simulink model "DC_microgrid_sliding_mode_control_NIKHIL_TYAGI"  (R2023b)
settings: Solver=VariableStepAuto  StartTime=0.0  StopTime=5  RelTol=1e-3
undefined symbols (not defined in the file): Ion, Lithium
libraries: spsFirstOrderFilterLib x19, spsCurrentMeasurementLib x11, spsSeriesRLCBranchLib x10, spsIGBTDiodeLib x4, spsVoltageMeasurementLib x4, spsPWMGeneratorDCDCLib x3, slpidlib x2, spsStairGeneratorLib x2, spsBatteryLib x1, spsDiodeLib x1, spsGroundLib x1, spsIGBTLib x1
settings Model: Creator=tyagi  LastModifiedBy=tyagi_av27qbo
settings OptimizationCC: ReuseModelBlockBuffer=off

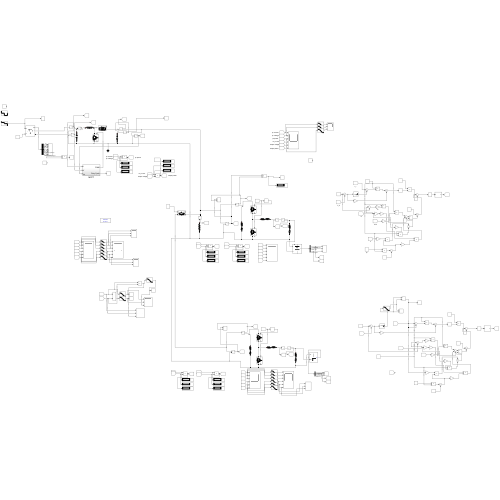
[thumbnail: Simulink's stored preview of the top-level diagram]
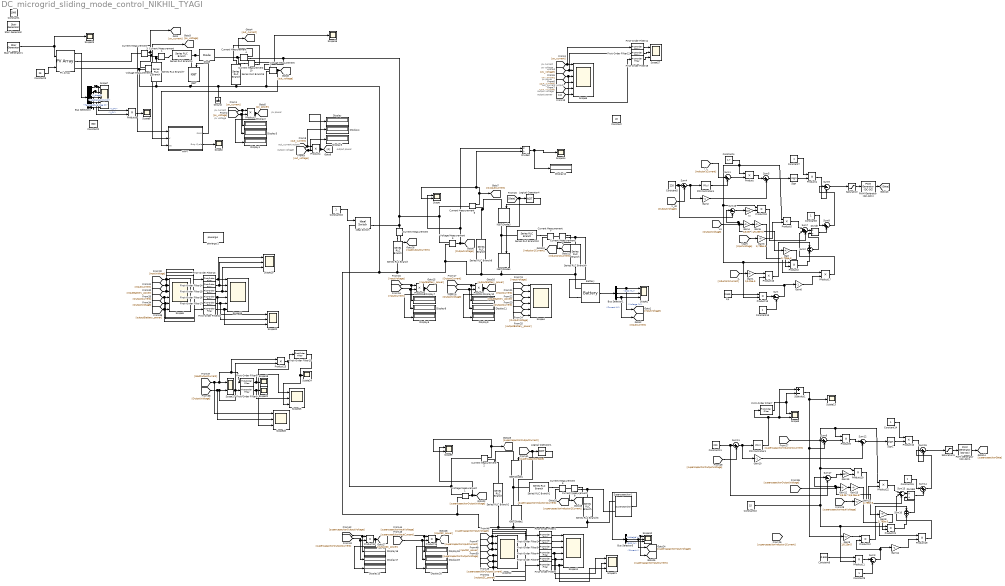
== system DC_microgrid_sliding_mode_control_NIKHIL_TYAGI ==
  note: pv power
  note: pv current
  note: out_current output
  note: pv voltage
  note: output voltage
  note: out_current output
  note: pv voltage
  note: pv power
  note: output voltage
  note: pv current
  note: output power
  note: output power
  Battery : spsBatteryLib/Battery  BatType=Lithium-Ion  ShowTempParam=off  ThermalPreset=no  ShowAgeParam=off  NomV=150  NomQ=15  SOC=100  Batt_Tr=30  PresetModel=on  MaxQ=15  MinV=112.5  FullV=174.5981  Dis_rate=6.5217  R=0.1  Normal_OP=13.5652  expZone="[162.0579     0.7369565]"  current=[6.5 13 32.5]  Units=Time  Tci=20  NomT=20  T2=-30  MaxQ2=4.8  FullV2=7.1  Normal_OP2=5.655  expZone2="[6.58           1]"  Rca=0.6  ti=2000  Dp=0  Neq0=0  Tsim=1e6  Ta1=25  Qeol=5.4*0.9  Reol=0.013333*1.2  Char_age=[2.3478, 3]  Dis_age=[2.3478, 10]  N1=1500  N2=10500  N3=1000  N4=1400  Ta2=45  N5=950
  Bus Selector1 : BusSelector  OutputSignals=Voltage (V),SOC (%),Current (A)
  Bus Selector2 : BusSelector  OutputSignals=V_PV,I_PV,I_diode,Irradiance (W/m2),Temperature (deg C)
  Bus Selector5 : BusSelector  OutputSignals=Current I,Voltage V,SOC %
  Constant : Constant  Value=40
  Constant1 : Constant  Value=1000
  Constant10 : Constant  Value=15
  Constant11 : Constant  Value=220
  Constant{7..9,13..16} (7 alike) : Constant
  Constant2 : Constant  Value=800
  Constant3 : Constant  Value=25
  Constant4 : Constant  Value=1.7
  Constant5 : Constant  Value=220
  Constant6 : Constant  Value=0.646
  Current Measurement{,1..10} (11 alike) : spsCurrentMeasurementLib/Current Measurement  PhasorSimulation=off  OutputType=Complex  PSBequivalent=0
  Diode : spsDiodeLib/Diode  Ron=0.001  Lon=0  Vf=0.8  IC=0  UseSnubber=0  Rs=500  Cs=250e-9  Measurements=on
  Display{,1..12,15..20} (19 alike) : Display
  Divide : Product  Inputs=*/
  Divide1 : Product  Inputs=*/
  Divide2 : Product  Inputs=*/
  First-Order Filter{1..6,8..19} (18 alike) : spsFirstOrderFilterLib/First-Order Filter  FilterType=Lowpass  Tc=10e-3  Ts=0  Initialize=on  Vac_Init=[0, 0, 60]  Vdc_Init=0  PlotResponse=off  FreqRange="[0,  200,  1]"
  First-Order Filter7 : spsFirstOrderFilterLib/First-Order Filter  FilterType=Lowpass  Tc=10e-3  Ts=0  Initialize=on  Vac_Init=[0, 0, 0]  Vdc_Init=0  PlotResponse=off  FreqRange="[0,  200,  1]"
  From13 : From
  Gain{,3,8,11} (4 alike) : Gain  Gain=1/.795e-3
  Gain1 : Gain  Gain=1/5.25e-5
  Gain{2,6,10,14} (4 alike) : Gain  Gain=-1
  Gain12 : Gain  Gain=1/8.06
  Gain13 : Gain  Gain=(1/5.25e-5)
  Gain15 : Gain  Gain=227
  Gain4 : Gain  Gain=1/8.06
  Gain5 : Gain  Gain=(1/5.25e-5)
  Gain9 : Gain  Gain=1/5.25e-5
  Goto9 : Goto
  Ground : spsGroundLib/Ground  LConnTagsString=a
  IGBT : spsIGBTLib/IGBT  Ron=0.001  Lon=0  Vf=1  Tf=1e-6  Tt=2e-6  IC=0  Rs=1e5  Cs=inf  Measurements=on
  IGBT/Diode{1..4} (4 alike) : spsIGBTDiodeLib/IGBT//Diode  Ron=1e-3  Rs=1e5  Cs=inf  Measurements=on
  Ideal Switch : spsIdealSwitchLib/Ideal Switch  Ron=0.001  Lon=0  IC=0  Rs=1e5  Cs=inf  Measurements=on
  Ki : Gain  Gain=227
  Kp : Constant  Value=0.646
  Logical Operator1 : Logic  Operator=NOT  AllPortsSameDT=off  OutDataTypeStr=boolean
  Logical Operator4 : Logic  Operator=NOT  AllPortsSameDT=off  OutDataTypeStr=boolean
  MPPT : Subsystem
  PID Controller1 : slpidlib/PID Controller  Controller=PI  Form=Parallel  TimeDomain=Continuous-time  UseExternalTs=off  SampleTime=-1  IntegratorMethod=Forward Euler  FilterMethod=Forward Euler  ControllerParametersSource=internal  P=0.646  I=227  UseKiTs=off  D=0  N=100  UseFilter=on  TunerSelectOption=Transfer Function Based (PID Tuner App)  InitialConditionSource=internal  InitialConditionForIntegrator=0  InitialConditionForFilter=0  DifferentiatorICPrevScaledInput=0  ExternalReset=none  TrackingMode=off  Kt=1  LimitOutput=on  SatLimitsSource=internal  UpperSaturationLimit=45  LowerSaturationLimit=0  LinearizeAsGain=on  AntiWindupMode=none  Kb=1  LimitIntegrator=off  UpperIntegratorSaturationLimit=inf  LowerIntegratorSaturationLimit=-inf  POutMin=[]  POutMax=[]  IOutMin=[]  IOutMax=[]  DOutMin=[]  DOutMax=[]  NOutMin=[]  NOutMax=[]  SumOutMin=[]  SumOutMax=[]  SaturationOutMin=[]  SaturationOutMax=[]  PParamMin=[]  PParamMax=[]  IParamMin=[]  IParamMax=[]  DParamMin=[]  DParamMax=[]  NParamMin=[]  NParamMax=[]  KbParamMin=[]  KbParamMax=[]  KtParamMin=[]  KtParamMax=[]  KbOutMin=[]  KbOutMax=[]  KtOutMin=[]  KtOutMax=[]  IntegratorOutMin=[]  IntegratorOutMax=[]  FilterOutMin=[]  FilterOutMax=[]  SumI1OutMin=[]  SumI1OutMax=[]  SumI2OutMin=[]  SumI2OutMax=[]  SumI3OutMin=[]  SumI3OutMax=[]  SumI4OutMin=[]  SumI4OutMax=[]  SumDOutMin=[]  SumDOutMax=[]  DifferentiatorOutMin=[]  DifferentiatorOutMax=[]  FilterDiffOutCoefMin=[]  FilterDiffOutCoefMax=[]  ReciprocalOutMin=[]  ReciprocalOutMax=[]  SumDenOutMin=[]  SumDenOutMax=[]  SumNumOutMin=[]  SumNumOutMax=[]  DivideOutMin=[]  DivideOutMax=[]  UdiffTsProdOutMin=[]  UdiffTsProdOutMax=[]  NTsProdOutMin=[]  NTsProdOutMax=[]  UintegralTsProdOutMin=[]  UintegralTsProdOutMax=[]  UngainTsProdOutMin=[]  UngainTsProdOutMax=[]  ClampingZeroOutDataTypeStr=Inherit: Inherit via back propagation  ClampingZeroOutMin=[]  ClampingZeroOutMax=[]  FilterDenConstantOutDataTypeStr=Inherit: Inherit via back propagation  FilterDenConstantOutMin=[]  FilterDenConstantOutMax=[]  PCopyOutDataTypeStr=Inherit: Inherit via back propagation  PCopyOutMin=[]  PCopyOutMax=[]  NCopyOutDataTypeStr=Inherit: Inherit via back propagation  NCopyOutMin=[]  NCopyOutMax=[]  IntegratorContinuousStateAttributes=''  IntegratorStateMustResolveToSignalObject=off  IntegratorRTWStateStorageClass=Auto  FilterContinuousStateAttributes=''  FilterStateMustResolveToSignalObject=off  FilterRTWStateStorageClass=Auto  ParallelPVariant=InternalParameters  IdealPVariant=Disabled  IVariant=InternalParameters  DVariant=Disabled  IntegratorVariant=Continuous  SatVariant=Enabled  AWVariant=Passthrough  PCopyVariant=Disabled  TRVariant=Disabled  FdbkBlocksVariant=Forward  IdealPFdbkVariant=Disabled  SatFdbkVariant=Disabled  DerivativeFilterVariant=Disabled  NVariant=Disabled  NCopyVariant=Disabled_SignalSpec  FilterICVariant=Disabled  IntegratorICVariant=InternalICs  ExternalResetVariant=Disabled  TRSumVariant=Passthrough  SumFdbkVariant=Disabled  SumVariant=Sum_PI  TsampFilterVariant=InternalTs  TsampNgainVariant=Passthrough  TsampIntegralVariant=Disabled_SignalSpec  ExternalSaturationOutDataTypeStr=Inherit: Same as second input
  PID Controller4 : slpidlib/PID Controller  Controller=PI  Form=Parallel  TimeDomain=Continuous-time  UseExternalTs=off  SampleTime=-1  IntegratorMethod=Forward Euler  FilterMethod=Forward Euler  ControllerParametersSource=internal  P=0.646  I=227  UseKiTs=off  D=0  N=100  UseFilter=on  TunerSelectOption=Transfer Function Based (PID Tuner App)  InitialConditionSource=internal  InitialConditionForIntegrator=0  InitialConditionForFilter=0  DifferentiatorICPrevScaledInput=0  ExternalReset=none  TrackingMode=off  Kt=1  LimitOutput=on  SatLimitsSource=internal  UpperSaturationLimit=45  LowerSaturationLimit=0  LinearizeAsGain=on  AntiWindupMode=none  Kb=1  LimitIntegrator=off  UpperIntegratorSaturationLimit=inf  LowerIntegratorSaturationLimit=-inf  POutMin=[]  POutMax=[]  IOutMin=[]  IOutMax=[]  DOutMin=[]  DOutMax=[]  NOutMin=[]  NOutMax=[]  SumOutMin=[]  SumOutMax=[]  SaturationOutMin=[]  SaturationOutMax=[]  PParamMin=[]  PParamMax=[]  IParamMin=[]  IParamMax=[]  DParamMin=[]  DParamMax=[]  NParamMin=[]  NParamMax=[]  KbParamMin=[]  KbParamMax=[]  KtParamMin=[]  KtParamMax=[]  KbOutMin=[]  KbOutMax=[]  KtOutMin=[]  KtOutMax=[]  IntegratorOutMin=[]  IntegratorOutMax=[]  FilterOutMin=[]  FilterOutMax=[]  SumI1OutMin=[]  SumI1OutMax=[]  SumI2OutMin=[]  SumI2OutMax=[]  SumI3OutMin=[]  SumI3OutMax=[]  SumI4OutMin=[]  SumI4OutMax=[]  SumDOutMin=[]  SumDOutMax=[]  DifferentiatorOutMin=[]  DifferentiatorOutMax=[]  FilterDiffOutCoefMin=[]  FilterDiffOutCoefMax=[]  ReciprocalOutMin=[]  ReciprocalOutMax=[]  SumDenOutMin=[]  SumDenOutMax=[]  SumNumOutMin=[]  SumNumOutMax=[]  DivideOutMin=[]  DivideOutMax=[]  UdiffTsProdOutMin=[]  UdiffTsProdOutMax=[]  NTsProdOutMin=[]  NTsProdOutMax=[]  UintegralTsProdOutMin=[]  UintegralTsProdOutMax=[]  UngainTsProdOutMin=[]  UngainTsProdOutMax=[]  ClampingZeroOutDataTypeStr=Inherit: Inherit via back propagation  ClampingZeroOutMin=[]  ClampingZeroOutMax=[]  FilterDenConstantOutDataTypeStr=Inherit: Inherit via back propagation  FilterDenConstantOutMin=[]  FilterDenConstantOutMax=[]  PCopyOutDataTypeStr=Inherit: Inherit via back propagation  PCopyOutMin=[]  PCopyOutMax=[]  NCopyOutDataTypeStr=Inherit: Inherit via back propagation  NCopyOutMin=[]  NCopyOutMax=[]  IntegratorContinuousStateAttributes=''  IntegratorStateMustResolveToSignalObject=off  IntegratorRTWStateStorageClass=Auto  FilterContinuousStateAttributes=''  FilterStateMustResolveToSignalObject=off  FilterRTWStateStorageClass=Auto  ParallelPVariant=InternalParameters  IdealPVariant=Disabled  IVariant=InternalParameters  DVariant=Disabled  IntegratorVariant=Continuous  SatVariant=Enabled  AWVariant=Passthrough  PCopyVariant=Disabled  TRVariant=Disabled  FdbkBlocksVariant=Forward  IdealPFdbkVariant=Disabled  SatFdbkVariant=Disabled  DerivativeFilterVariant=Disabled  NVariant=Disabled  NCopyVariant=Disabled_SignalSpec  FilterICVariant=Disabled  IntegratorICVariant=InternalICs  ExternalResetVariant=Disabled  TRSumVariant=Passthrough  SumFdbkVariant=Disabled  SumVariant=Sum_PI  TsampFilterVariant=InternalTs  TsampNgainVariant=Passthrough  TsampIntegralVariant=Disabled_SignalSpec  ExternalSaturationOutDataTypeStr=Inherit: Same as second input
  PV Array : spsPVArrayLib/PV Array  Npar=8  Nser=2  PlotType=array @ 25 deg.C & specified irradiances  S_vec="[ 1000  500  100 ]"  Temp_C_vec="[ 45 25  ]"  ModuleName=SunPower SPR-E19-310-COM  PlotWhenSelected=off  Pm=310.149  Ncell=96  Voc=64.4  Isc=6.05  Vm=54.7  Im=5.67  beta_Voc_pc=-0.2727  alpha_Isc_pc=0.061736  beta_Voc=-0.17562  alpha_Isc=0.003735  IL=6.0753  I0=6.4157e-12  nI=0.94792  Rsh=341.5455  Rs=0.40157  RobustModel=off  RobustCellTemperature=313.3991  BAL=off  Tc=1e-6  Tfilter=5e-5
  PWM Generator (DC-DC)1 : spsPWMGeneratorDCDCLib/PWM Generator (DC-DC)  Fsw=15000  Ts=0
  PWM Generator (DC-DC)2 : spsPWMGeneratorDCDCLib/PWM Generator (DC-DC)  Fsw=15000  Ts=0
  Product{,1..23} (24 alike) : Product
  Saturation : Saturate  UpperLimit=1  LowerLimit=0
  Saturation1 : Saturate  UpperLimit=1  LowerLimit=0
  Scope{,3,9,17} (4 alike) : Scope  NumInputPorts=2
  Scope{1,10,19..21,25,27..28} (8 alike) : Scope  NumInputPorts=3
  Scope{4..6,11..12,15} (6 alike) : Scope  NumInputPorts=6
  Scope{2,8,13..14,16,18,22..24} (9 alike) : Scope
  Scope7 : Scope  NumInputPorts=5
  Series RLC Branch : spsSeriesRLCBranchLib/Series RLC Branch  LConnTagsString=__new0  RConnTagsString=__new0  BranchType=R  Resistance=8.06  Inductance=1e-3  SetiL0=off  InitialCurrent=0  Capacitance=1e-6  Setx0=off  InitialVoltage=0  Measurements=None
  Series RLC Branch1 : spsSeriesRLCBranchLib/Series RLC Branch  LConnTagsString=__new0  RConnTagsString=__new0  BranchType=RL  Resistance=0.0001  Inductance=.795e-3  SetiL0=off  InitialCurrent=0  Capacitance=1e-6  Setx0=off  InitialVoltage=0  Measurements=None
  Series RLC Branch10 : spsSeriesRLCBranchLib/Series RLC Branch  LConnTagsString=__new0  RConnTagsString=__new0  BranchType=RL  Resistance=0.0001  Inductance=.795e-3  SetiL0=off  InitialCurrent=0  Capacitance=1e-6  Setx0=off  InitialVoltage=0  Measurements=None
  Series RLC Branch2 : spsSeriesRLCBranchLib/Series RLC Branch  LConnTagsString=__new0  RConnTagsString=__new0  BranchType=RC  Resistance=.0001  Inductance=1e-3  SetiL0=off  InitialCurrent=0  Capacitance=1000e-6  Setx0=off  InitialVoltage=0  Measurements=None
  Series RLC Branch3 : spsSeriesRLCBranchLib/Series RLC Branch  LConnTagsString=__new0  RConnTagsString=__new0  BranchType=RC  Resistance=0.0001  Inductance=1e-3  SetiL0=off  InitialCurrent=0  Capacitance=4.44e-6  Setx0=off  InitialVoltage=0  Measurements=None
  Series RLC Branch4 : spsSeriesRLCBranchLib/Series RLC Branch  LConnTagsString=__new0  RConnTagsString=__new0  BranchType=L  Resistance=1  Inductance=.336e-3  SetiL0=off  InitialCurrent=0  Capacitance=1e-6  Setx0=off  InitialVoltage=0  Measurements=None
  Series RLC Branch6 : spsSeriesRLCBranchLib/Series RLC Branch  LConnTagsString=__new0  RConnTagsString=__new0  BranchType=C  Resistance=0.001  Inductance=1e-3  SetiL0=off  InitialCurrent=0  Capacitance=4000.31e-6  Setx0=off  InitialVoltage=0  Measurements=None
  Series RLC Branch7 : spsSeriesRLCBranchLib/Series RLC Branch  LConnTagsString=__new0  RConnTagsString=__new0  BranchType=C  Resistance=1e-3  Inductance=1e-3  SetiL0=off  InitialCurrent=0  Capacitance=1000e-6  Setx0=off  InitialVoltage=0  Measurements=None
  Series RLC Branch8 : spsSeriesRLCBranchLib/Series RLC Branch  LConnTagsString=__new0  RConnTagsString=__new0  BranchType=RC  Resistance=.0001  Inductance=1e-3  SetiL0=off  InitialCurrent=0  Capacitance=1000e-6  Setx0=off  InitialVoltage=0  Measurements=None
  Series RLC Branch9 : spsSeriesRLCBranchLib/Series RLC Branch  LConnTagsString=__new0  RConnTagsString=__new0  BranchType=RC  Resistance=0.0001  Inductance=1e-3  SetiL0=off  InitialCurrent=0  Capacitance=4.44e-6  Setx0=off  InitialVoltage=0  Measurements=None
  Sign : Signum
  Sign1 : Signum
  Stair Generator : spsStairGeneratorLib/Stair Generator  t=[0, 1, 3, 5]  e=[1, .8, .6,.8]*1000  Ts=0
  Stair Generator1 : spsStairGeneratorLib/Stair Generator  t=[0, 1, 3, 5]  e=[1, .8, .6,.2]*1000  Ts=0
  Subtract1 : Sum  Inputs=+-
  Sum{,1,3..4,6,9,11,15..17} (10 alike) : Sum  Inputs=|+-
  Sum10 : Sum
  Sum{5,8,12,14} (4 alike) : Sum  Inputs=|++
  Sum13 : Sum  Inputs=|-++
  Sum2 : Sum
  Sum7 : Sum  Inputs=|-++
  Supercapacitor1 : spsSupercapacitorLib/Supercapacitor  C=30  Rdc=8.9e-3  Voltage=300  Ns=100  Np=2  Vinit=200  Temp=25  PresetModel=off  EstParam=off  Nc=1  r=1e-9  epsilon=6.0208e-10  Ich=10  Vstern="[0.161  2.7  7.8]"  Self_dis=on  Ioc=10  Vself="[48  47.8  47.06  44.65]"  demandeplot=off  I="[10  20 100  500]"  Units=sec  Vmax=0  If=0  deltaV=0  alpha=0  sec=0
      settings: LibrarySourceBlock=sps_lib/Sources/Supercapacitor
  Voltage Measurement{1..3,5} (4 alike) : spsVoltageMeasurementLib/Voltage Measurement  PhasorSimulation=off  OutputType=Complex  PSBequivalent=0
  powergui1 : spspowerguiLib/powergui  Priority=1  SimulationMode=Discrete  SampleTime=50e-6  frequency=60  Iterations=50  frequencyindice=0  Pbase=100e6  ErrMax=1e-4  UnitsV=kV  UnitsW=MW  buscounter=0  FunctionMessages=off  echomessages=off  EnableUseOfTLC=off  CurrentSourceSwitches=off  DisableSnubberDevices=off  DisableRonSwitches=off  DisableVfSwitches=off  DisplayEquations=off  AutomaticDiscreteSolvers=off  SolverType=Tustin/Backward Euler (TBE)  Interpol=off  ExternalGateDelay=off  methode=off  Ts=100  x0status=blocks  SPID=on  SwTol=0  HookPort=off  NonlinearTolerance=1e-4  nMaxIteration=100  ContinueOnMaxIteration=off  RestoreLinks=warning  ResistiveCurrentMeasurement=off  Frange=[0:2:500]  Ylog=off  Xlog=on  ShowGrid=off  save=off  variable=ZData  structure=0  ZoomFFT=off  StartTime=0.0  cycles=1  DisplayStyle=1  fundamental=60  FreqAxis=off  MaxFrequency=1000  frequencyindicesteady=1  RmsSteady=1  display=off
  wires:
  Gain3/1 -> Product5/2
  Sum8/1 -> Sum9/1
  [InputVoltage] -> Gain3/1
  Constant8/1 -> Sum8/1
  Current Measurement6/1 -> Divide2/2, Scope/2, [OutputCurrent]
  [OutputVoltage] -> Sum4/2
  Current Measurement7/1 -> [Inductor1Current]
  Sum7/1 -> Divide/1
  Constant4/1 -> Product5/1, Product18/1, Product13/2, Product2/1, Product/1
  Bus Selector1/3 -> [InputCurrent], Scope1/3  "<Current (A)>"
  Constant5/1 -> Sum16/2, Sum4/1
  PID Controller4/1 -> Sum1/2
  PWM Generator (DC-DC)2/1 -> [Gate]
  Gain2/1 -> Sum5/2
  Sign/1 -> Product1/2
  [Inductor1Current] -> Sum1/1
  Product/1 -> Sum5/1
  Current Measurement9/1 -> [Inductor2Current]
  Product5/1 -> Sum7/1
  Gain4/1 -> Gain5/1
  [OutputVoltage] -> Display11/1, Product8/2
  Product1/1 -> Sum9/2
  Sum9/1 -> Saturation/1
  [InputCurrent] -> Scope4/2
  [InputVoltage] -> Display7/1, Product7/1
  Voltage Measurement5/1 -> Divide2/1, Scope/1, [OutputVoltage]
  Sum1/1 -> Product/2
  [InputCurrent] -> Display8/1, Product7/2
  [Gate] -> IGBT/Diode4/1, Logical Operator4/1
  Logical Operator4/1 -> IGBT/Diode3/1
  Divide/1 -> Sum8/2
  [Inductor1Current] -> Gain1/1
  Sum2/1 -> Divide/2
  Product7/1 -> Display6/1, [inputBattery_power]
  Battery/1 -> Bus Selector1/1
  Bus Selector1/2 -> Scope1/2  "<SOC (%)>"
  Current Measurement/1 -> [loadOutputCurrent]
  Product2/1 -> Sum2/2
  [outputBattery_power] -> Scope4/6
  [OutputVoltage] -> Scope4/5
  [OutputCurrent] -> Display10/1, Product8/1
  Sum5/1 -> Sign/1
  Gain5/1 -> Product17/1
  Gain1/1 -> Product16/1
  Sum4/1 -> Gain2/1, PID Controller4/1
  [OutputCurrent] -> Scope4/4
  Constant7/1 -> Product1/1
  Product8/1 -> Display9/1, [outputBattery_power]
  [InputVoltage] -> Scope4/1
  [inputBattery_power] -> Scope4/3
  Bus Selector1/1 -> [InputVoltage], Scope1/1  "<Voltage (V)>"
  Gain/1 -> Product2/2
  MPPT/1(PWM) -> IGBT/1
  Voltage Measurement3/1 -> [pv_voltage], MPPT/2(V)
  Bus Selector2/3 -> Scope7/3  "<I_diode>"
  Voltage Measurement2/1 -> MPPT/3(Vo), [out_voltage]
  Current Measurement3/1 -> MPPT/1(I), [pv_current]
  [pv_current] -> First-Order Filter11/1, Scope5/1
  Product6/1 -> Scope8/1
  Bus Selector2/4 -> Scope7/4  "<Irradiance (W/m2)>"
  [pv_current] -> Display2/1, Product3/1
  [out_voltage] -> Scope5/5
  [out_current] -> Display4/1, Product4/1
  Bus Selector2/2 -> Product6/2, Scope7/2  "<I_PV>"
  Current Measurement10/1 -> Scope16/1
  [pv_voltage] -> First-Order Filter12/1, Scope5/2
  PV Array/1 -> Bus Selector2/1
  [out_current] -> Scope5/4
  [out_voltage] -> Display5/1, Product4/2
  [pv_power] -> First-Order Filter19/1, Scope5/3
  Constant3/1 -> PV Array/2
  [pv_voltage] -> Display3/1, Product3/2
  MPPT/2(Duty Cycle) -> Scope2/1
  Bus Selector2/1 -> Product6/1, Scope7/1  "<V_PV>"
  From13/1 -> Scope5/6
  Stair Generator1/1 -> Scope23/1, PV Array/1
  Product4/1 -> Display/1, Goto9/1
  Product3/1 -> Display1/1, [pv_power]
  Current Measurement4/1 -> [out_current]
  Bus Selector2/5 -> Scope7/5  "<Temperature (deg C)>"
  Product16/1 -> Sum2/1
  [OutputVoltage] -> Gain/1, Gain4/1, Sum16/1
  Product18/1 -> Sum7/3
  [supercapacitorInputVoltage] -> Display18/1, Product15/1
  Product14/1 -> Display15/1, [outputSC_power]
  [supercapacitorOutputCurrent] -> First-Order Filter5/1, Scope12/5
  [OutputVoltage] -> First-Order Filter17/1, Scope6/5
  First-Order Filter16/1 -> Scope20/1, Scope15/4
  Logical Operator1/1 -> IGBT/Diode1/1
  [supercapacitorGate] -> IGBT/Diode2/1, Logical Operator1/1
  [outputSC_power] -> First-Order Filter6/1, Scope12/6
  First-Order Filter18/1 -> Scope20/3, Scope15/6
  First-Order Filter14/1 -> Scope19/2, Scope15/2
  First-Order Filter13/1 -> Scope19/1, Scope15/1
  First-Order Filter15/1 -> Scope19/3, Scope15/3
  Current Measurement5/1 -> [supercapacitorInductor1Current]
  First-Order Filter5/1 -> Scope11/5, Scope21/2
  First-Order Filter17/1 -> Scope20/2, Scope15/5
  First-Order Filter4/1 -> Scope21/1, Scope11/4
  First-Order Filter6/1 -> Scope21/3, Scope11/6
  [supercapacitorOutputCurrent] -> Display17/1, Product14/2
  First-Order Filter3/1 -> Scope11/3
  Bus Selector5/2 -> [supercapacitorInputVoltage], Scope10/2  "<Voltage V>"
  Product15/1 -> Display20/1, [inputSC_power]
  First-Order Filter2/1 -> Scope11/2
  Bus Selector5/3 -> Scope10/3  "<SOC %>"
  Current Measurement2/1 -> Scope9/2, [supercapacitorOutputCurrent]
  [supercapacitorInputCurrent] -> First-Order Filter2/1, Scope12/2
  [inputSC_power] -> First-Order Filter3/1, Scope12/3
  [InputVoltage] -> First-Order Filter13/1, Scope6/1
  Current Measurement8/1 -> [supercapacitorInductor2Current]
  [supercapacitorOutputVoltage] -> Display16/1, Product14/1
  [inputBattery_power] -> First-Order Filter15/1, Scope6/3
  [supercapacitorOutputVoltage] -> First-Order Filter4/1, Scope12/4
  [supercapacitorInputCurrent] -> Display19/1, Product15/2
  Bus Selector5/1 -> [supercapacitorInputCurrent], Scope10/1  "<Current I>"
  [InputCurrent] -> First-Order Filter14/1, Scope6/2
  [supercapacitorInputVoltage] -> First-Order Filter1/1, Scope12/1
  Supercapacitor1/1 -> Bus Selector5/1
  [OutputCurrent] -> Scope6/4, First-Order Filter16/1
  [outputBattery_power] -> First-Order Filter18/1, Scope6/6
  First-Order Filter1/1 -> Scope11/1
  Voltage Measurement1/1 -> Scope9/1, [supercapacitorOutputVoltage]
  Kp/1 -> Product13/1
  Product13/1 -> Sum/1
  Constant13/1 -> Sum/2
  Sum/1 -> Gain6/1, Product16/2
  Gain6/1 -> Product17/2
  Product17/1 -> Sum7/2
  Ki/1 -> Product18/2
  Saturation/1 -> PWM Generator (DC-DC)2/1
  PID Controller1/1 -> First-Order Filter7/1, Subtract1/1, Scope3/2
  First-Order Filter7/1 -> Scope3/1, Subtract1/2
  Product12/1 -> Sum10/1
  Constant9/1 -> Sum3/2
  Product11/1 -> Sum3/1
  Sum3/1 -> Gain14/1, Product12/2
  Product20/1 -> Sum13/3
  Gain14/1 -> Product19/2
  Saturation1/1 -> PWM Generator (DC-DC)1/1
  Sum15/1 -> Saturation1/1
  PWM Generator (DC-DC)1/1 -> [supercapacitorGate]
  Divide1/1 -> Sum14/2
  Product9/1 -> Sum12/1
  Gain11/1 -> Product22/2
  Gain10/1 -> Sum12/2
  Product19/1 -> Sum13/2
  Subtract1/1 -> Gain9/1, Sum6/2, Scope13/1
  Constant14/1 -> Product10/1
  Product22/1 -> Sum13/1
  Gain15/1 -> Product20/2
  Sum6/1 -> Product9/2
  Constant10/1 -> Product22/1, Product9/1, Product20/1, Product11/2, Product21/1
  Sum13/1 -> Divide1/1
  [supercapacitorOutputVoltage] -> Sum17/1, Gain8/1, Gain12/1
  Gain9/1 -> Product12/1
  Sum11/1 -> Gain10/1, PID Controller1/1
  Gain13/1 -> Product19/1
  Sum10/1 -> Divide1/2
  Gain8/1 -> Product21/2
  Product21/1 -> Sum10/2
  Gain12/1 -> Gain13/1
  Sum14/1 -> Sum15/1
  Constant11/1 -> Sum17/2, Sum11/1
  [supercapacitorOutputVoltage] -> Sum11/2
  Sign1/1 -> Product10/2
  Product10/1 -> Sum15/2
  [supercapacitorInputVoltage] -> Gain11/1
  Constant15/1 -> Sum14/1
  Constant6/1 -> Product11/1
  [supercapacitorInductor1Current] -> Sum6/1
  Sum12/1 -> Sign1/1
  Divide2/1 -> Display12/1, Scope14/1
  Sum16/1 -> Ki/1
  Sum17/1 -> Gain15/1
  [OutputVoltage] -> Scope28/2, Product23/2, First-Order Filter9/1, Scope17/2
  [loadOutputCurrent] -> Scope28/1, Product23/1, First-Order Filter8/1, Scope17/1
  First-Order Filter9/1 -> Scope25/2, Scope22/1
  First-Order Filter8/1 -> Scope25/1, Scope18/1
  Constant16/1 -> Ideal Switch/1
  First-Order Filter10/1 -> Scope25/3, Scope24/1
  Product23/1 -> Scope28/3, First-Order Filter10/1
  First-Order Filter11/1 -> Scope27/1
  First-Order Filter12/1 -> Scope27/2
  First-Order Filter19/1 -> Scope27/3
  connections:
  Battery/LConn1 -- Series RLC Branch9/LConn1 -- Current Measurement9/RConn1
  Series RLC Branch2/RConn1 -- Voltage Measurement2/LConn2 -- Series RLC Branch6/RConn1 -- Ground/LConn1 -- IGBT/RConn1 -- Series RLC Branch7/RConn1 -- Voltage Measurement3/LConn2 -- PV Array/RConn2 -- Voltage Measurement5/LConn2 -- Series RLC Branch8/RConn1 -- Battery/LConn2 -- Series RLC Branch9/RConn1 -- IGBT/Diode4/RConn1 -- Series RLC Branch/RConn1 -- Voltage Measurement1/LConn2 -- IGBT/Diode2/RConn1 -- Series RLC Branch3/RConn1 -- Supercapacitor1/LConn2
  IGBT/Diode4/LConn1 -- IGBT/Diode3/RConn1 -- Series RLC Branch10/LConn1
  Voltage Measurement2/LConn1 -- Current Measurement4/RConn1 -- Voltage Measurement5/LConn1 -- Current Measurement6/LConn1 -- Ideal Switch/RConn1 -- Current Measurement/LConn1
  IGBT/Diode3/LConn1 -- Series RLC Branch8/LConn1 -- Current Measurement6/RConn1
  Current Measurement9/LConn1 -- Current Measurement7/LConn1
  Current Measurement/RConn1 -- Series RLC Branch/LConn1
  Series RLC Branch10/RConn1 -- Current Measurement7/RConn1
  Current Measurement3/RConn1 -- Voltage Measurement3/LConn1 -- Current Measurement1/LConn1 -- Series RLC Branch7/LConn1
  Current Measurement10/LConn1 -- Current Measurement4/LConn1 -- Diode/RConn1
  Series RLC Branch4/RConn1 -- IGBT/LConn1 -- Diode/LConn1
  PV Array/RConn1 -- Current Measurement3/LConn1
  Current Measurement1/RConn1 -- Series RLC Branch4/LConn1
  Current Measurement10/RConn1 -- Series RLC Branch6/LConn1
  Series RLC Branch3/LConn1 -- Current Measurement8/RConn1 -- Supercapacitor1/LConn1
  IGBT/Diode1/LConn1 -- Current Measurement2/RConn1 -- Series RLC Branch2/LConn1
  IGBT/Diode2/LConn1 -- IGBT/Diode1/RConn1 -- Series RLC Branch1/LConn1
  Series RLC Branch1/RConn1 -- Current Measurement5/RConn1
  Current Measurement8/LConn1 -- Current Measurement5/LConn1
  Current Measurement2/LConn1 -- Voltage Measurement1/LConn1 -- Ideal Switch/LConn1

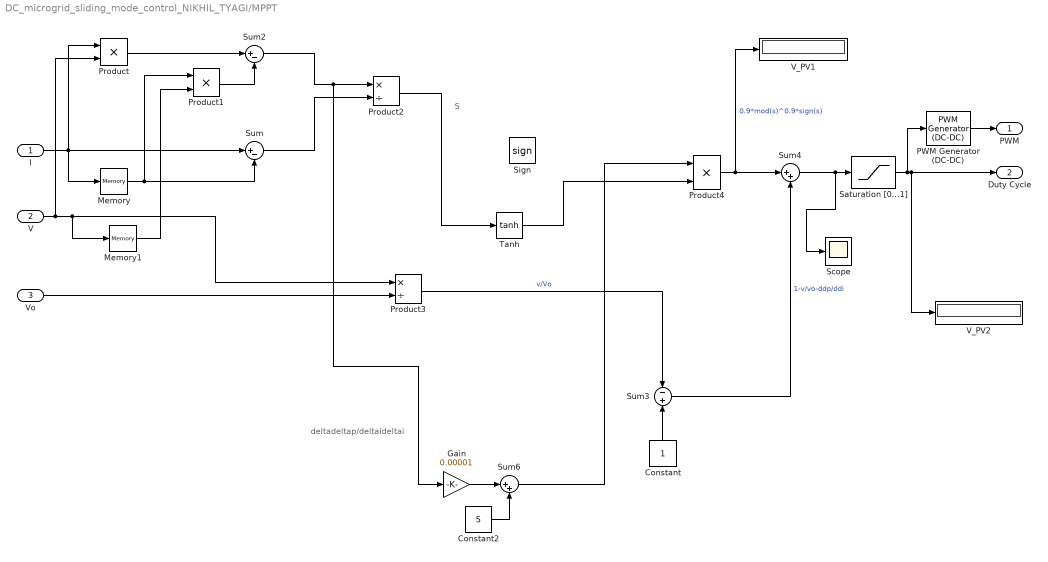
== system DC_microgrid_sliding_mode_control_NIKHIL_TYAGI/MPPT ==
  note: deltadeltap/deltaideltai
  note: S
  I : Inport
  V : Inport  Port=2
  Vo : Inport  Port=3
  Constant : Constant
  Constant2 : Constant  Value=5
  Gain : Gain  Gain=0.00001
  Memory : Memory  InheritSampleTime=on
  Memory1 : Memory  InheritSampleTime=on
  PWM Generator (DC-DC) : spsPWMGeneratorDCDCLib/PWM Generator (DC-DC)  Fsw=10000  Ts=0
  Product : Product
  Product1 : Product
  Product2 : Product  Inputs=*/
  Product3 : Product  Inputs=*/
  Product4 : Product
  Saturation [0...1] : Saturate  UpperLimit=1  LowerLimit=0
  Scope : Scope
  Sign : Signum  ZeroCross=off
  Sum : Sum  Inputs=|+-
  Sum2 : Sum  Inputs=|+-
  Sum3 : Sum  Inputs=-|+
  Sum4 : Sum  Inputs=|++
  Sum6 : Sum  Inputs=|++
  Tanh : Trigonometry  Operator=tanh
  V_PV1 : Display
  V_PV2 : Display
  PWM : Outport
  Duty Cycle : Outport  Port=2
  wires:
  I/1 -> Memory/1, Product/1, Sum/1
  Memory/1 -> Sum/2, Product1/1
  V/1 -> Product3/1, Memory1/1, Product/2
  Memory1/1 -> Product1/2
  Product/1 -> Sum2/1
  Product1/1 -> Sum2/2
  Sum/1 -> Product2/2
  Sum2/1 -> Gain/1, Product2/1
  Vo/1 -> Product3/2
  Product3/1 -> Sum3/1  "v/Vo"
  Sum6/1 -> Product4/1
  Product4/1 -> V_PV1/1, Sum4/1  "0.9*mod(s)^0.9*sign(s)"
  PWM Generator (DC-DC)/1 -> PWM/1
  Saturation [0...1]/1 -> V_PV2/1, Duty Cycle/1, PWM Generator (DC-DC)/1
  Sum4/1 -> Scope/1, Saturation [0...1]/1
  Constant/1 -> Sum3/2
  Sum3/1 -> Sum4/2  "1-v/vo-ddp/ddi"
  Gain/1 -> Sum6/1
  Constant2/1 -> Sum6/2
  Product2/1 -> Tanh/1
  Tanh/1 -> Product4/2
